simulink library "Tire_Parts_235_80R17"  (R2022a)
settings: Solver=VariableStepAuto  StartTime=0.0  StopTime=10.0  RelTol=1e-3
undefined symbols (not defined in the file): X, Y, Z
libraries: sm_lib x7, $bdroot x4
Description:
  | Copyright 2020-2023 The MathWorks, Inc.
settings Model: Creator=smiller  LastModifiedBy=smiller
settings SolverCC: AlgebraicLoopSolver=TrustRegion
settings DataIOCC: ReturnWorkspaceOutputs=off
settings DebuggingCC: UnconnectedInputMsg=warning  UnconnectedOutputMsg=warning  UnconnectedLineMsg=warning  ArithmeticOperatorsInVariantConditions=warning
settings SFSimCC: CustomCodeUndefinedFunction=UseInterfaceOnly

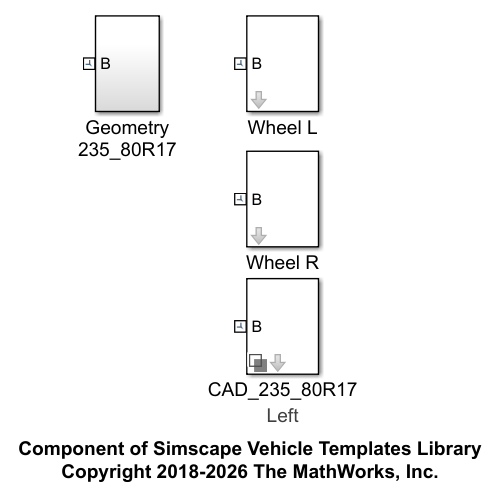
[thumbnail: Simulink's stored preview of the top-level diagram]
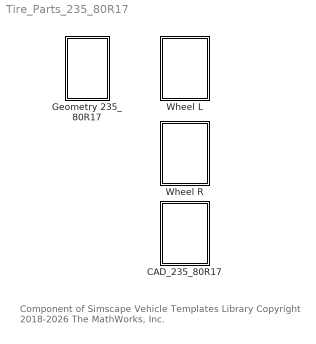
== system Tire_Parts_235_80R17 ==
  note: Component of Simscape Vehicle Templates Library
      | Copyright 2018-2026 The MathWorks, Inc.
  CAD_235_80R17 : Subsystem  Variant=on  VariantControlMode=label  LabelModeActiveChoice=Left  mask(Wheel Geometry, Mass, Inertia){popup_leftRight=Left, mass_tire=10, mass_rim=0, tire_inertia=[1 2], rim_inertia=[0 0], offset_cg=[0 0 0]}
      mask prompts: popup_leftRight "Left/Right"; offset_cg "CG Offset [x y z] (m)"
      mask help: Models geometry, mass, and inertia for tire size 235 80R17 (single tire). Drop down selects left or right side.
      mask init:
      | set_param(gcb,'LabelModeActiveChoice',get_param(gcb,'popup_LeftRight'));
      settings: AttributesFormatString=%<LabelModeActiveChoice>
      mask TypeOptions popup_leftRight: Left | Right
      mask DialogControl text_tire Prompt: Tire
      mask DialogControl text_rim Prompt: Rim
      mask DialogControl text_mass Prompt: Mass (kg)
      mask DialogControl text_inertia Prompt: Inertia [Ixx Iyy] (kg*m^2)
      mask Display: disp(' ');
  Geometry 235_80R17 : Subsystem
  Wheel L : Subsystem  mask(Wheel Geometry, Mass, Inertia){mass_tire=10, mass_rim=0, tire_inertia=[1 2], rim_inertia=[0 0], offset_cg=[0 0 0]}
      mask prompts: offset_cg "CG Offset [x y z] (m)"
      mask help: Models geometry, mass, and inertia for tire size 235 80R17 (left side).
      mask init:
      | Imat = [tire_inertia(1)+rim_inertia(1) 0 0; 0 tire_inertia(1)+rim_inertia(1) 0; 0 0 tire_inertia(2)+rim_inertia(2)];
      | wheel_mass = mass_tire + mass_rim;
      mask DialogControl text_tire Prompt: Tire
      mask DialogControl text_rim Prompt: Rim
      mask DialogControl text_mass Prompt: Mass (kg)
      mask DialogControl text_inertia Prompt: Inertia [Ixx Iyy] (kg*m^2)
  Wheel R : Subsystem  mask(Wheel Geometry, Mass, Inertia){mass_tire=10, mass_rim=0, tire_inertia=[1 2], rim_inertia=[0 0], offset_cg=[0 0 0]}
      mask prompts: offset_cg "CG Offset [x y z] (m)"
      mask help: Models geometry, mass, and inertia for tire size 235 80R17 (right side).
      mask init:
      | Imat = [tire_inertia(1)+rim_inertia(1) 0 0; 0 tire_inertia(1)+rim_inertia(1) 0; 0 0 tire_inertia(2)+rim_inertia(2)];
      | wheel_mass = mass_tire + mass_rim;
      mask DialogControl text_tire Prompt: Tire
      mask DialogControl text_rim Prompt: Rim
      mask DialogControl text_mass Prompt: Mass (kg)
      mask DialogControl text_inertia Prompt: Inertia [Ixx Iyy] (kg*m^2)

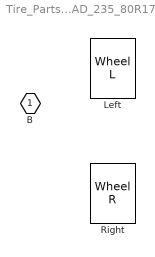
== system Tire_Parts_235_80R17/CAD_235_80R17 ==
  Left : $bdroot/Wheel L  VariantControl=Left  mass_tire=mass_tire  mass_rim=mass_rim  tire_inertia=tire_inertia  rim_inertia=rim_inertia  offset_cg=offset_cg
  Right : $bdroot/Wheel R  VariantControl=Right  mass_tire=mass_tire  mass_rim=mass_rim  tire_inertia=tire_inertia  rim_inertia=rim_inertia  offset_cg=offset_cg
  B : PMIOPort  Side=Left

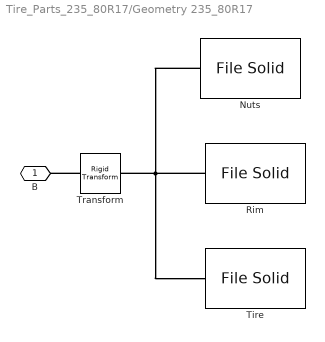
== system Tire_Parts_235_80R17/Geometry 235_80R17 ==
  Nuts : sm_lib/Body Elements/File Solid  ExtGeomFileName=SUV_Landy_Whl_Nuts.stl  UnitType=Custom  ExtGeomFileUnits=m  StepReaderType=HEX  ExportConvexHullGeometry=off  InertiaType=PointMass  Mass=0  MassUnits=kg  CenterOfMass=[0 0 0]  CenterOfMassUnits=m  MomentsOfInertia=[1 1 1]  MomentsOfInertiaUnits=kg*m^2  ProductsOfInertia=[0 0 0]  ProductsOfInertiaUnits=kg*m^2  BasedOnType=Density  Density=1000  DensityUnits=kg/m^3  DoExposeReferenceFrame=on  SerializedFrames=<Frames/>  GraphicType=FromGeometry  MarkerShape=Sphere  MarkerSize=10  GraphicVisPropType=SimpleVisualProperties  GraphicDiffuseColor=[0.489721, 0.438681, 0.438681]  GraphicSpecularColor=[0.5 0.5 0.5 1.0]  GraphicAmbientColor=[0.15 0.15 0.15 1.0]  GraphicEmissiveColor=[0.0 0.0 0.0 1.0]  GraphicShininess=75  GraphicOpacity=1.000000
  Rim : sm_lib/Body Elements/File Solid  ExtGeomFileName=SUV_Landy_Whl_Rim.stl  UnitType=Custom  ExtGeomFileUnits=m  StepReaderType=HEX  ExportConvexHullGeometry=off  InertiaType=PointMass  Mass=0  MassUnits=kg  CenterOfMass=[0 0 0]  CenterOfMassUnits=m  MomentsOfInertia=[1 1 1]  MomentsOfInertiaUnits=kg*m^2  ProductsOfInertia=[0 0 0]  ProductsOfInertiaUnits=kg*m^2  BasedOnType=Density  Density=1000  DensityUnits=kg/m^3  DoExposeReferenceFrame=on  SerializedFrames=<Frames/>  GraphicType=FromGeometry  MarkerShape=Sphere  MarkerSize=10  GraphicVisPropType=SimpleVisualProperties  GraphicDiffuseColor=[0.634436, 0.643989, 0.682236]  GraphicSpecularColor=[0.5 0.5 0.5 1.0]  GraphicAmbientColor=[0.15 0.15 0.15 1.0]  GraphicEmissiveColor=[0.0 0.0 0.0 1.0]  GraphicShininess=75  GraphicOpacity=1.000000
  Tire : sm_lib/Body Elements/File Solid  ExtGeomFileName=SUV_Landy_Whl_Tire.stl  UnitType=Custom  ExtGeomFileUnits=m  StepReaderType=HEX  ExportConvexHullGeometry=off  InertiaType=PointMass  Mass=0  MassUnits=kg  CenterOfMass=[0 0 0]  CenterOfMassUnits=m  MomentsOfInertia=[1 1 1]  MomentsOfInertiaUnits=kg*m^2  ProductsOfInertia=[0 0 0]  ProductsOfInertiaUnits=kg*m^2  BasedOnType=Density  Density=1000  DensityUnits=kg/m^3  DoExposeReferenceFrame=on  SerializedFrames=<Frames/>  GraphicType=FromGeometry  MarkerShape=Sphere  MarkerSize=10  GraphicVisPropType=SimpleVisualProperties  GraphicDiffuseColor=[0.280667, 0.284494, 0.299801]  GraphicSpecularColor=[0.5 0.5 0.5 1.0]  GraphicAmbientColor=[0.15 0.15 0.15 1.0]  GraphicEmissiveColor=[0.0 0.0 0.0 1.0]  GraphicShininess=75  GraphicOpacity=1.000000
  Transform : sm_lib/Frames and Transforms/Rigid Transform  TranslationMethod=None  TranslationStandardOffset=0  TranslationLengthUnit=m  TranslationStandardAxis=+Z  TranslationCartesianOffset=[0 0 0]  TranslationROffset=0  TranslationROffsetUnits=m  TranslationZOffset=0  TranslationZOffsetUnits=m  TranslationThetaOffset=0  TranslationThetaOffsetUnits=deg  RotationMethod=StandardAxis  RotationAngleUnits=deg  RotationStandardAxis=+X  RotationAngle=90  RotationArbitraryAxis=[0 0 1]  FollAlignAxisA=+X  BaseAlignAxisA=+Y  FollAlignAxisB=+Y  BaseAlignAxisB=+Z  RotationSequenceAxes=FollowerAxes  RotationSequence=XYX  RotationSequenceAngles=[0 0 0]  RotationSequenceAnglesUnits=deg  RotationMatrix=[1 0 0;0 1 0;0 0 1]
  B : PMIOPort  Side=Left
  connections:
  Nuts/RConn1 -- Transform/RConn1 -- Tire/RConn1 -- Rim/RConn1
  Transform/LConn1 -- B/RConn1

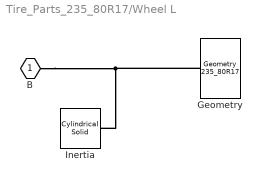
== system Tire_Parts_235_80R17/Wheel L ==
  Geometry : $bdroot/Geometry 235_80R17  SystemSampleTime=-1  VariantActivationTime=update diagram  Latency=0  AutoFrameSizeCalculation=off
  Inertia : sm_lib/Body Elements/Cylindrical Solid  GraphicAmbientColor=[0.15 0.15 0.15 1.0]  BasedOnType=Density  CenterOfMass=offset_cg  CenterOfMassUnits=m  GraphicDiffuseColor=[0.2 0.8 1.0]  CylinderLength=0.001  CylinderLengthUnits=m  CylinderRadius=0.001  CylinderRadiusUnits=m  Density=1000  DensityUnits=kg/(m^3)  DoExposeReferenceFrame=on  GraphicEmissiveColor=[0.0 0.0 0.0 1.0]  ExportEntireGeometry=off  SerializedFrames=<Frames/>  MarkerShape=Sphere  MarkerSize=10  GraphicType=FromGeometry  InertiaType=Custom  Mass=wheel_mass  MassUnits=kg  MomentsOfInertia=[Imat(1,1) Imat(2,2) Imat(3,3)]  MomentsOfInertiaUnits=kg*m^2  GraphicOpacity=1.0  ProductsOfInertia=[0 0 0]  ProductsOfInertiaUnits=kg*m^2  GraphicShininess=75  GraphicSpecularColor=[0.5 0.5 0.5 1.0]  GraphicVisPropType=SimpleVisualProperties
  B : PMIOPort  Side=Left
  connections:
  B/RConn1 -- Geometry/LConn1 -- Inertia/RConn1

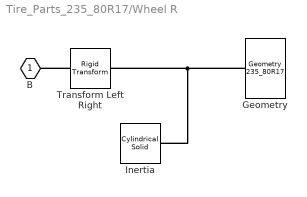
== system Tire_Parts_235_80R17/Wheel R ==
  Geometry : $bdroot/Geometry 235_80R17  SystemSampleTime=-1  VariantActivationTime=update diagram  Latency=0  AutoFrameSizeCalculation=off
  Inertia : sm_lib/Body Elements/Cylindrical Solid  GraphicAmbientColor=[0.15 0.15 0.15 1.0]  BasedOnType=Density  CenterOfMass=offset_cg  CenterOfMassUnits=m  GraphicDiffuseColor=[0.2 0.8 1.0]  CylinderLength=0.001  CylinderLengthUnits=m  CylinderRadius=0.001  CylinderRadiusUnits=m  Density=1000  DensityUnits=kg/(m^3)  DoExposeReferenceFrame=on  GraphicEmissiveColor=[0.0 0.0 0.0 1.0]  ExportEntireGeometry=off  SerializedFrames=<Frames/>  MarkerShape=Sphere  MarkerSize=10  GraphicType=FromGeometry  InertiaType=Custom  Mass=wheel_mass  MassUnits=kg  MomentsOfInertia=[Imat(1,1) Imat(2,2) Imat(3,3)]  MomentsOfInertiaUnits=kg*m^2  GraphicOpacity=1.0  ProductsOfInertia=[0 0 0]  ProductsOfInertiaUnits=kg*m^2  GraphicShininess=75  GraphicSpecularColor=[0.5 0.5 0.5 1.0]  GraphicVisPropType=SimpleVisualProperties
  Transform Left Right : sm_lib/Frames and Transforms/Rigid Transform  TranslationMethod=None  TranslationStandardOffset=0  TranslationLengthUnit=m  TranslationStandardAxis=+Z  TranslationCartesianOffset=[0 0 0]  TranslationROffset=0  TranslationROffsetUnits=m  TranslationZOffset=0  TranslationZOffsetUnits=m  TranslationThetaOffset=0  TranslationThetaOffsetUnits=deg  RotationMethod=StandardAxis  RotationAngleUnits=deg  RotationStandardAxis=+X  RotationAngle=180  RotationArbitraryAxis=[0 0 1]  FollAlignAxisA=+X  BaseAlignAxisA=+Y  FollAlignAxisB=+Y  BaseAlignAxisB=+Z  RotationSequenceAxes=FollowerAxes  RotationSequence=XYX  RotationSequenceAngles=[0 0 0]  RotationSequenceAnglesUnits=deg  RotationMatrix=[1 0 0; 0 1 0; 0 0 1]
  B : PMIOPort  Side=Left
  connections:
  Transform Left Right/RConn1 -- Geometry/LConn1 -- Inertia/RConn1
  Transform Left Right/LConn1 -- B/RConn1
